simulink model "gs_vector_test"  (R2016b)
settings: Solver=VariableStepAuto  StartTime=0.0  StopTime=6400  RelTol=1e-3
values from neighbouring files (symbols this model uses):
  fsw_params = init_fsw_params()    [gs_vector_test_init.m]
libraries: gps x1, gs_prediction_lib x1, sgp4_lib_fsw x1, teme_2_eci_lib x1, time_coord_rotation_lib x1
settings Model: Creator=Taylor  LastModifiedBy=taylorreynolds

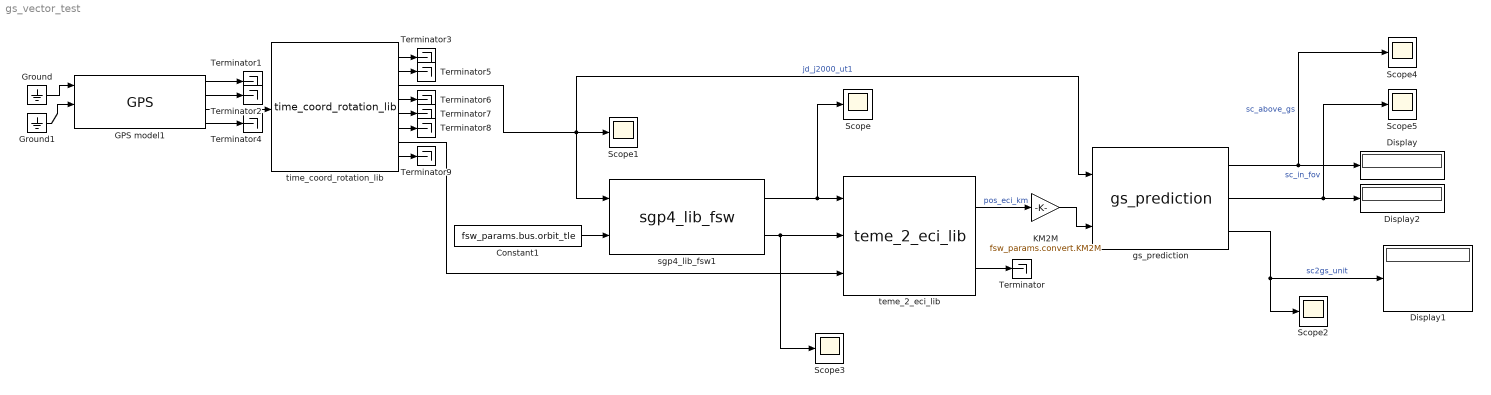
== system gs_vector_test ==
  Constant1 : Constant  Value=fsw_params.bus.orbit_tle
  Display : Display
  Display1 : Display
  Display2 : Display
  GPS model1 : gps/GPS
  Ground : Ground
  Ground1 : Ground
  KM2M : Gain  Gain=fsw_params.convert.KM2M
  Scope{,1..5} (6 alike) : Scope
  Terminator{,1..9} (10 alike) : Terminator
  gs_prediction : gs_prediction_lib/gs_prediction
  sgp4_lib_fsw1 : sgp4_lib_fsw/sgp4_lib_fsw
  teme_2_eci_lib : teme_2_eci_lib/teme_2_eci_lib
  time_coord_rotation_lib : time_coord_rotation_lib/time_coord_rotation_lib
  wires:
  gs_prediction/1 -> Display/1, Scope4/1  "sc_above_gs"
  gs_prediction/3 -> Scope2/1, Display1/1  "sc2gs_unit"
  sgp4_lib_fsw1/1 -> Scope/1, teme_2_eci_lib/1
  sgp4_lib_fsw1/2 -> Scope3/1, teme_2_eci_lib/2
  teme_2_eci_lib/1 -> KM2M/1  "pos_eci_km"
  teme_2_eci_lib/2 -> Terminator/1
  time_coord_rotation_lib/3 -> gs_prediction/1, Scope1/1, sgp4_lib_fsw1/1  "jd_j2000_ut1"
  time_coord_rotation_lib/7 -> teme_2_eci_lib/3
  Constant1/1 -> sgp4_lib_fsw1/2
  KM2M/1 -> gs_prediction/2
  time_coord_rotation_lib/1 -> Terminator3/1
  GPS model1/1 -> Terminator1/1
  GPS model1/2 -> Terminator2/1
  GPS model1/4 -> Terminator4/1
  Ground1/1 -> GPS model1/2
  Ground/1 -> GPS model1/1
  gs_prediction/2 -> Scope5/1, Display2/1  "sc_in_fov"
  GPS model1/3 -> time_coord_rotation_lib/1
  time_coord_rotation_lib/2 -> Terminator5/1
  time_coord_rotation_lib/4 -> Terminator6/1
  time_coord_rotation_lib/5 -> Terminator7/1
  time_coord_rotation_lib/6 -> Terminator8/1
  time_coord_rotation_lib/8 -> Terminator9/1
